simulink model "fourier_series_32"  (R2018a)
settings: Solver=VariableStepAuto  StartTime=0.0  StopTime=2  RelTol=1e-3
libraries: simulink x2
settings Model: Creator=barne  LastModifiedBy=weishij2

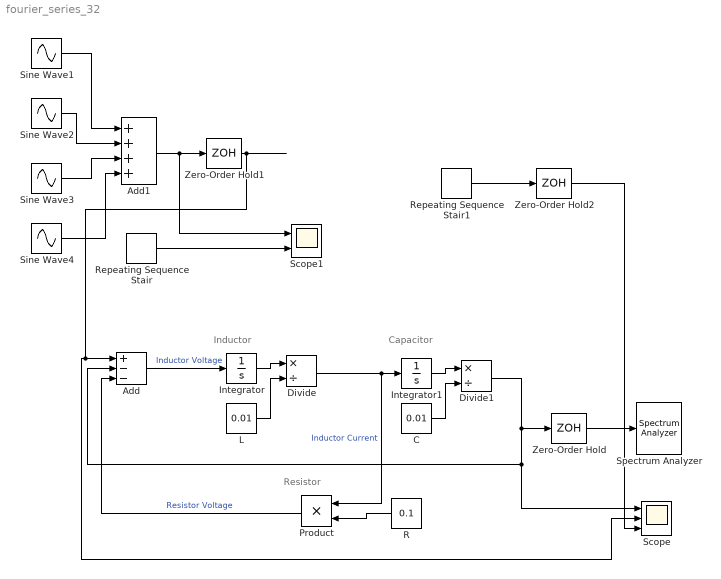
== system fourier_series_32 ==
  note: Resistor
  note: Inductor
  note: Capacitor
  Add : Sum  Inputs=+--
  Add1 : Sum  Inputs=++++
  C : Constant  Value=0.01
  Divide : Product  Inputs=*/
  Divide1 : Product  Inputs=*/
  Integrator : Integrator
  Integrator1 : Integrator
  L : Constant  Value=0.01
  Product : Product
  R : Constant  Value=0.1
  Repeating Sequence Stair : simulink/Sources/Repeating Sequence Stair  OutValues=[-1 1]  tsamp=1/64  OutMin=[]  OutMax=[]  OutDataTypeStr=double  OutputDataTypeScalingMode=double  OutDataType=fixdt(0,8)  ConRadixGroup=Best Precision: Vector-wise  OutScaling=2^-12
  Repeating Sequence Stair1 : simulink/Sources/Repeating Sequence Stair  OutValues=[1 -1]  tsamp=1/64  OutMin=[]  OutMax=[]  OutDataTypeStr=double  OutputDataTypeScalingMode=double  OutDataType=fixdt(0,8)  ConRadixGroup=Best Precision: Vector-wise  OutScaling=2^-12
  Scope : Scope  NumInputPorts=3
  Scope1 : Scope  NumInputPorts=2
  Sine Wave1 : Sin  Amplitude=(4/pi)*(1/1)  Frequency=2*pi*1*32  SampleTime=0
  Sine Wave2 : Sin  Amplitude=(4/pi)*(1/3)  Frequency=2*pi*3*32  SampleTime=0
  Sine Wave3 : Sin  Amplitude=(4/pi)*(1/5)  Frequency=2*pi*5*32  SampleTime=0
  Sine Wave4 : Sin  Amplitude=(4/pi)*(1/4)  Frequency=2*pi*4*32  SampleTime=0
  Spectrum Analyzer : SpectrumAnalyzer
  Zero-Order Hold : ZeroOrderHold  SampleTime=2^(-10)
  Zero-Order Hold1 : ZeroOrderHold  SampleTime=2^(-10)
  Zero-Order Hold2 : ZeroOrderHold  SampleTime=2^(-10)
  wires:
  Add/1 -> Integrator/1  "Inductor Voltage"
  Integrator/1 -> Divide/1
  L/1 -> Divide/2
  Divide/1 -> Product/1, Integrator1/1  "Inductor Current"
  Integrator1/1 -> Divide1/1
  C/1 -> Divide1/2
  R/1 -> Product/2
  Product/1 -> Add/3  "Resistor Voltage"
  Divide1/1 -> Add/2, Scope/1, Zero-Order Hold/1
  Zero-Order Hold/1 -> Spectrum Analyzer/1
  Zero-Order Hold1/1 -> Scope/2, Add/1
  Sine Wave2/1 -> Add1/2
  Sine Wave4/1 -> Add1/4
  Sine Wave3/1 -> Add1/3
  Add1/1 -> Scope1/1, Zero-Order Hold1/1
  Repeating Sequence Stair/1 -> Scope1/2
  Sine Wave1/1 -> Add1/1
  Zero-Order Hold2/1 -> Scope/3
  Repeating Sequence Stair1/1 -> Zero-Order Hold2/1
